simulink model "Spring_Mass2_Damper"  (R2019a)
settings: Solver=VariableStepAuto  StartTime=0.0  StopTime=10  RelTol=1e-3
values from neighbouring files (symbols this model uses):
  C = 1    [value.m]
  K = 1    [value.m]
  M1 = 1    [value.m]
  M2 = 1    [value.m]
settings Model: Creator=Takumi SHIOTA  LastModifiedBy=Takumi SHIOTA

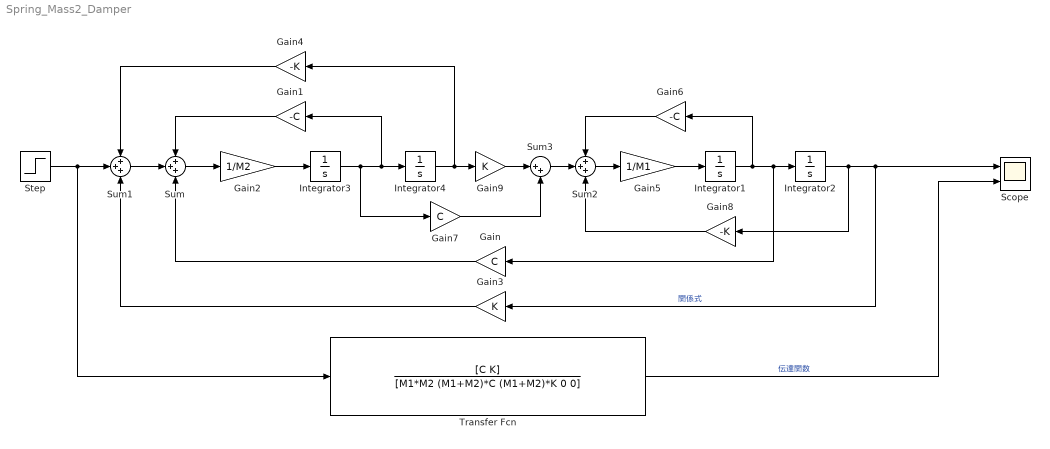
== system Spring_Mass2_Damper ==
  Gain : Gain  Gain=C
  Gain1 : Gain  Gain=-C
  Gain2 : Gain  Gain=1/M2
  Gain3 : Gain  Gain=K
  Gain4 : Gain  Gain=-K
  Gain5 : Gain  Gain=1/M1
  Gain6 : Gain  Gain=-C
  Gain7 : Gain  Gain=C
  Gain8 : Gain  Gain=-K
  Gain9 : Gain  Gain=K
  Integrator{1..4} (4 alike) : Integrator
  Scope : Scope  NumInputPorts=2
  Step : Step  SampleTime=0
  Sum : Sum  Inputs=+++
  Sum1 : Sum  Inputs=+++
  Sum2 : Sum  Inputs=+++
  Sum3 : Sum  Inputs=|++
  Transfer Fcn : TransferFcn  Numerator=[C K]  Denominator=[M1*M2 (M1+M2)*C (M1+M2)*K 0 0]
  wires:
  Integrator3/1 -> Integrator4/1, Gain1/1, Gain7/1
  Integrator1/1 -> Integrator2/1, Gain/1, Gain6/1
  Integrator2/1 -> Scope/1, Gain3/1, Gain8/1  "関係式"
  Sum/1 -> Gain2/1
  Step/1 -> Sum1/2, Transfer Fcn/1
  Gain2/1 -> Integrator3/1
  Transfer Fcn/1 -> Scope/2  "伝達関数"
  Gain/1 -> Sum/3
  Gain1/1 -> Sum/1
  Gain3/1 -> Sum1/3
  Sum1/1 -> Sum/2
  Gain4/1 -> Sum1/1
  Gain6/1 -> Sum2/1
  Sum2/1 -> Gain5/1
  Gain8/1 -> Sum2/3
  Sum3/1 -> Sum2/2
  Integrator4/1 -> Gain9/1, Gain4/1
  Gain5/1 -> Integrator1/1
  Gain9/1 -> Sum3/1
  Gain7/1 -> Sum3/2
